simulink model "simulink2"  (R2016a)
settings: Solver=ode5  StartTime=0.0  StopTime=30.0  FixedStep=0.01  RelTol=1e-3
settings Model: Creator=Abhay  LastModifiedBy=Abhay
settings DataIOCC: LimitDataPoints=on  SaveFormat=Array
settings DebuggingCC: SolverPrmCheckMsg=warning
settings HardwareCC: ProdBitPerPointer=32  ProdLargestAtomicFloat=None  ProdIntDivRoundTo=Undefined  ProdEndianess=Unspecified  ProdWordSize=32  ProdHWDeviceType=32-bit Generic
settings ModelReferenceCC: PropagateSignalLabelsOutOfModel=off
settings ConfigComp: CovModelRefEnable=Off  CovSFcnEnable=off

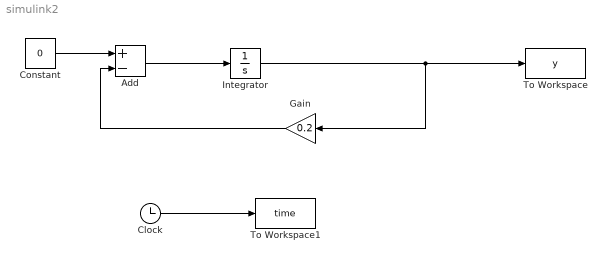
== system simulink2 ==
  Add : Sum  Inputs=+-
  Clock : Clock
  Constant : Constant  Value=0
  Gain : Gain  Gain=0.2
  Integrator : Integrator
  To Workspace : ToWorkspace  VariableName=y  SampleTime=-1
  To Workspace1 : ToWorkspace  VariableName=time  SampleTime=-1
  wires:
  Clock/1 -> To Workspace1/1
  Constant/1 -> Add/1
  Add/1 -> Integrator/1
  Integrator/1 -> Gain/1, To Workspace/1
  Gain/1 -> Add/2
